simulink library "MinSegLibrary_MinSegMega"  (R2015b)
settings: Solver=ode45  StartTime=0.0  StopTime=10.0  RelTol=1e-3
libraries: arduinolib x2
settings Model: Creator=hurstj  LastModifiedBy=Administrator
settings DataIOCC: SaveFormat=Array
settings DebuggingCC: UnderspecifiedInitializationDetection=Classic  MergeDetectMultiDrivingBlocksExec=none  SolverPrmCheckMsg=warning  StateNameClashWarn=warning
settings HardwareCC: ProdBitPerPointer=32  ProdLargestAtomicFloat=None  ProdIntDivRoundTo=Undefined  ProdEndianess=Unspecified  ProdWordSize=32  ProdHWDeviceType=32-bit Generic
settings GRTTargetCC: GeneratePreprocessorConditionals=Disable all
settings ConfigComp: CovModelRefEnable=Off

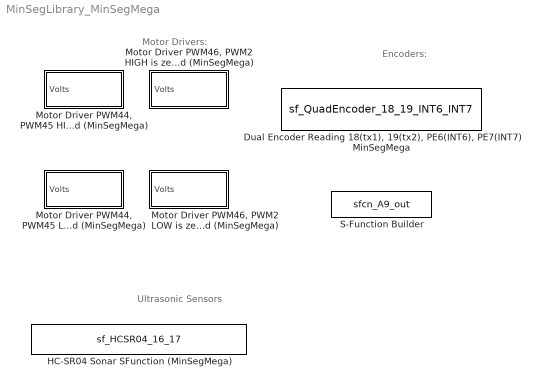
== system MinSegLibrary_MinSegMega ==
  note: Motor Drivers:
  note: Ultrasonic Sensors
  note: Encoders:
  "Dual Encoder Reading 18(tx1), 19(tx2), PE6(INT6), PE7(INT7) MinSegMega " : S-Function  InitFcn=try, set_param(gcb,'FunctionName','sf_QuadEncoder_18_19_INT6_INT7'), end  FunctionName=sf_QuadEncoder_18_19_INT6_INT7  Parameters=uint8([0 1]),uint8([18 6]),uint8([19 7])  SFunctionModules=sf_QuadEncoder_18_19_INT6_INT7_wrapper  SFunctionDeploymentMode=off  EnableBusSupport=off  mask(S-Function Builder){}
      mask init:
      | val = [[.9  0.75 0.75 1 1 .9 .9 1]',[1 1 0.75 0.75 .9 .9 1 .9]'];try , sys = get_param(gcb,'SfunBuilderFcnName');if isempty(sys), sys = get_param(gcb,'FunctionName'); end,catch, sys = get_param(gcb,'FunctionName'); end
      settings: CopyFcn=set_param(gcbh,'LinkStatus','none')  PreSaveFcn=try, set_param(gcb,'FunctionName','sf_QuadEncoder_18_19_INT6_INT7'), end  OpenFcn=sfunctionwizard(gcbh)
      mask Display: plot(val(:,1),val(:,2)),disp(sys), port_label('output',1,'pos1'), port_label('output',2,'pos2')
  HC-SR04 Sonar SFunction (MinSegMega) : S-Function  InitFcn=try, set_param(gcb,'FunctionName','sf_HCSR04_16_17'), end  FunctionName=sf_HCSR04_16_17  SFunctionModules=sf_HCSR04_16_17_wrapper  SFunctionDeploymentMode=off  EnableBusSupport=off  mask(S-Function Builder){}
      mask help: Simulink:masks:SFunctionBuilder_MD
      mask init: same as MinSegLibrary_MinSegMega/Dual Encoder Reading 18(tx1), 19(tx2), PE6(INT6), PE7(INT7) MinSegMega 
      settings: CopyFcn=set_param(gcbh,'LinkStatus','none')  PreSaveFcn=try, set_param(gcb,'FunctionName','sf_HCSR04_16_17'), end  OpenFcn=sfunctionwizard(gcbh)
      mask Display: plot(val(:,1),val(:,2)),disp(sys), port_label('output',1,'distance_cm')
  "Motor Driver PWM44, PWM45 HIGH is zero speed (MinSegMega)" : Subsystem
  "Motor Driver PWM44, PWM45 LOW is zero speed (MinSegMega)" : Subsystem
  "Motor Driver PWM46, PWM2 HIGH is zero speed (MinSegMega)" : Subsystem
  "Motor Driver PWM46, PWM2 LOW is zero speed (MinSegMega)" : Subsystem
  S-Function Builder : S-Function  InitFcn=try, set_param(gcb,'FunctionName','sfcn_A9_out'), end  FunctionName=sfcn_A9_out  Parameters=uint8(9)  SFunctionModules=sfcn_A9_out_wrapper  SFunctionDeploymentMode=off  EnableBusSupport=off  mask(S-Function Builder){}
      mask init: same as MinSegLibrary_MinSegMega/Dual Encoder Reading 18(tx1), 19(tx2), PE6(INT6), PE7(INT7) MinSegMega 
      settings: CopyFcn=set_param(gcbh,'LinkStatus','none')  PreSaveFcn=try, set_param(gcb,'FunctionName','sfcn_A9_out'), end  OpenFcn=sfunctionwizard(gcbh)
      mask Display: plot(val(:,1),val(:,2)),disp(sys), port_label('input',1,'in')

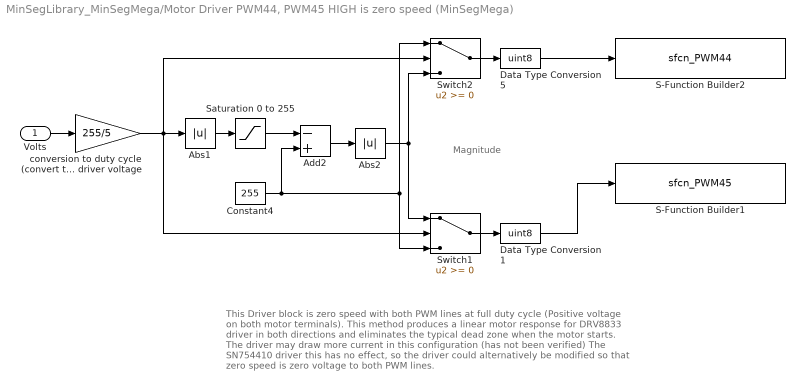
== system MinSegLibrary_MinSegMega/Motor Driver PWM44, PWM45 HIGH is zero speed (MinSegMega) ==
  note: Magnitude
  note: This Driver block is zero speed with both PWM lines at full duty cycle
      |  (Positive voltage on both motor terminals).
      | This method produces a linear motor response for DRV8833 driver
      |  in both directions and eliminates
      | the typical dead zone when the motor starts.
      | The driver may draw more current in this configuration (has not been verified)
      |
      | The SN754410 driver this has no effect, so the driver could alternatively
      | be modified so that zero speed is zero voltage to both PWM lines.
  Volts : Inport
  Abs1 : Abs
  Abs2 : Abs
  Add2 : Sum  Inputs=-+
  Constant4 : Constant  Value=255
  Data Type Conversion1 : DataTypeConversion  OutDataTypeStr=uint8
  Data Type Conversion5 : DataTypeConversion  OutDataTypeStr=uint8
  S-Function Builder1 : S-Function  InitFcn=try, set_param(gcb,'FunctionName','sfcn_PWM45'), end  FunctionName=sfcn_PWM45  Parameters=uint8(45)  SFunctionModules=sfcn_PWM45_wrapper  SFunctionDeploymentMode=off  EnableBusSupport=off  mask(S-Function Builder){}
      mask init: same as MinSegLibrary_MinSegMega/Dual Encoder Reading 18(tx1), 19(tx2), PE6(INT6), PE7(INT7) MinSegMega 
      settings: CopyFcn=set_param(gcbh,'LinkStatus','none')  PreSaveFcn=try, set_param(gcb,'FunctionName','sfcn_PWM45'), end  OpenFcn=sfunctionwizard(gcbh)
      mask Display: plot(val(:,1),val(:,2)),disp(sys), port_label('input',1,'in')
  S-Function Builder2 : S-Function  InitFcn=try, set_param(gcb,'FunctionName','sfcn_PWM44'), end  FunctionName=sfcn_PWM44  Parameters=uint8(44)  SFunctionModules=sfcn_PWM44_wrapper  SFunctionDeploymentMode=off  EnableBusSupport=off  mask(S-Function Builder){}
      mask init: same as MinSegLibrary_MinSegMega/Dual Encoder Reading 18(tx1), 19(tx2), PE6(INT6), PE7(INT7) MinSegMega 
      settings: CopyFcn=set_param(gcbh,'LinkStatus','none')  PreSaveFcn=try, set_param(gcb,'FunctionName','sfcn_PWM44'), end  OpenFcn=sfunctionwizard(gcbh)
      mask Display: plot(val(:,1),val(:,2)),disp(sys), port_label('input',1,'in')
  Saturation 0 to 255 : Saturate  UpperLimit=255  LowerLimit=0
  Switch1 : Switch
  Switch2 : Switch
  conversion to duty cycle (convert to int) denominator is motor driver voltage : Gain  Gain=255/5  OutDataTypeStr=int16
  wires:
  Data Type Conversion1/1 -> S-Function Builder1/1
  Data Type Conversion5/1 -> S-Function Builder2/1
  Switch1/1 -> Data Type Conversion1/1
  Switch2/1 -> Data Type Conversion5/1
  Abs2/1 -> Switch1/1, Switch2/3
  Add2/1 -> Abs2/1
  Constant4/1 -> Add2/2, Switch2/1, Switch1/3
  Abs1/1 -> Saturation 0 to 255/1
  Saturation 0 to 255/1 -> Add2/1
  conversion to duty cycle (convert to int) denominator is motor driver voltage/1 -> Switch1/2, Switch2/2, Abs1/1
  Volts/1 -> conversion to duty cycle (convert to int) denominator is motor driver voltage/1

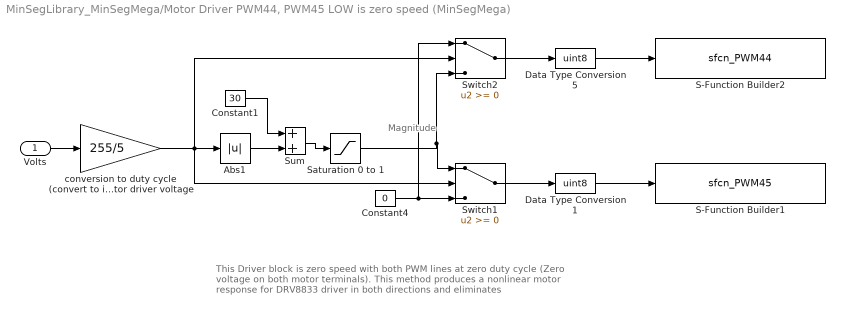
== system MinSegLibrary_MinSegMega/Motor Driver PWM44, PWM45 LOW is zero speed (MinSegMega) ==
  note: This Driver block is zero speed with both PWM lines at zero duty cycle
      |  (Zero voltage on both motor terminals).
      | This method produces a nonlinear motor response for DRV8833 driver
      |  in both directions and eliminates
  note: Magnitude
  Volts : Inport
  Abs1 : Abs
  Constant1 : Constant  Value=30
  Constant4 : Constant  Value=0
  Data Type Conversion1 : DataTypeConversion  OutDataTypeStr=uint8
  Data Type Conversion5 : DataTypeConversion  OutDataTypeStr=uint8
  S-Function Builder1 : S-Function  InitFcn=try, set_param(gcb,'FunctionName','sfcn_PWM45'), end  FunctionName=sfcn_PWM45  Parameters=uint8(45)  SFunctionModules=sfcn_PWM45_wrapper  SFunctionDeploymentMode=off  EnableBusSupport=off  mask(S-Function Builder){}
      mask init: same as MinSegLibrary_MinSegMega/Dual Encoder Reading 18(tx1), 19(tx2), PE6(INT6), PE7(INT7) MinSegMega 
      settings: CopyFcn=set_param(gcbh,'LinkStatus','none')  PreSaveFcn=try, set_param(gcb,'FunctionName','sfcn_PWM45'), end  OpenFcn=sfunctionwizard(gcbh)
      mask Display: plot(val(:,1),val(:,2)),disp(sys), port_label('input',1,'in')
  S-Function Builder2 : S-Function  InitFcn=try, set_param(gcb,'FunctionName','sfcn_PWM44'), end  FunctionName=sfcn_PWM44  Parameters=uint8(44)  SFunctionModules=sfcn_PWM44_wrapper  SFunctionDeploymentMode=off  EnableBusSupport=off  mask(S-Function Builder){}
      mask init: same as MinSegLibrary_MinSegMega/Dual Encoder Reading 18(tx1), 19(tx2), PE6(INT6), PE7(INT7) MinSegMega 
      settings: CopyFcn=set_param(gcbh,'LinkStatus','none')  PreSaveFcn=try, set_param(gcb,'FunctionName','sfcn_PWM44'), end  OpenFcn=sfunctionwizard(gcbh)
      mask Display: plot(val(:,1),val(:,2)),disp(sys), port_label('input',1,'in')
  Saturation 0 to 1 : Saturate  UpperLimit=255  LowerLimit=0
  Sum : Sum
  Switch1 : Switch
  Switch2 : Switch
  conversion to duty cycle (convert to int) denominator is motor driver voltage : Gain  Gain=255/5  OutDataTypeStr=int16
  wires:
  Volts/1 -> conversion to duty cycle (convert to int) denominator is motor driver voltage/1
  conversion to duty cycle (convert to int) denominator is motor driver voltage/1 -> Switch1/2, Abs1/1, Switch2/2
  Constant4/1 -> Switch2/1, Switch1/3
  Saturation 0 to 1/1 -> Switch2/3, Switch1/1
  Switch2/1 -> Data Type Conversion5/1
  Switch1/1 -> Data Type Conversion1/1
  Data Type Conversion5/1 -> S-Function Builder2/1
  Data Type Conversion1/1 -> S-Function Builder1/1
  Abs1/1 -> Sum/2
  Sum/1 -> Saturation 0 to 1/1
  Constant1/1 -> Sum/1

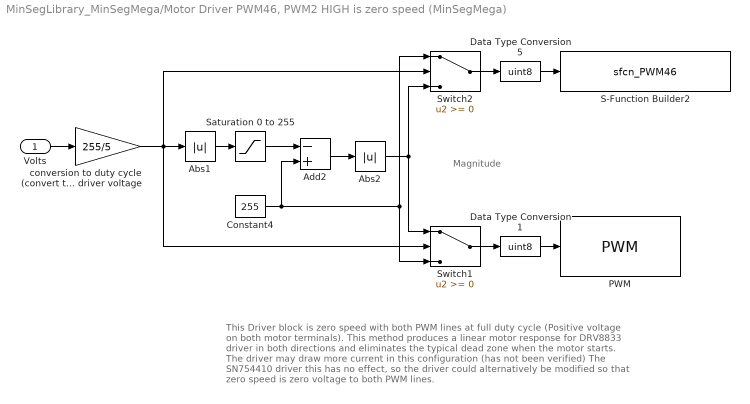
== system MinSegLibrary_MinSegMega/Motor Driver PWM46, PWM2 HIGH is zero speed (MinSegMega) ==
  note: Magnitude
  note: This Driver block is zero speed with both PWM lines at full duty cycle
      |  (Positive voltage on both motor terminals).
      | This method produces a linear motor response for DRV8833 driver
      |  in both directions and eliminates
      | the typical dead zone when the motor starts.
      | The driver may draw more current in this configuration (has not been verified)
      |
      | The SN754410 driver this has no effect, so the driver could alternatively
      | be modified so that zero speed is zero voltage to both PWM lines.
  Volts : Inport
  Abs1 : Abs
  Abs2 : Abs
  Add2 : Sum  Inputs=-+
  Constant4 : Constant  Value=255
  Data Type Conversion1 : DataTypeConversion  OutDataTypeStr=uint8
  Data Type Conversion5 : DataTypeConversion  OutDataTypeStr=uint8
  PWM : arduinolib/PWM  pinNumber=2
  S-Function Builder2 : S-Function  InitFcn=try, set_param(gcb,'FunctionName','sfcn_PWM46'), end  FunctionName=sfcn_PWM46  Parameters=uint8(46)  SFunctionModules=sfcn_PWM46_wrapper  SFunctionDeploymentMode=off  EnableBusSupport=off  mask(S-Function Builder){}
      mask init: same as MinSegLibrary_MinSegMega/Dual Encoder Reading 18(tx1), 19(tx2), PE6(INT6), PE7(INT7) MinSegMega 
      settings: CopyFcn=set_param(gcbh,'LinkStatus','none')  PreSaveFcn=try, set_param(gcb,'FunctionName','sfcn_PWM46'), end  OpenFcn=sfunctionwizard(gcbh)
      mask Display: plot(val(:,1),val(:,2)),disp(sys), port_label('input',1,'in')
  Saturation 0 to 255 : Saturate  UpperLimit=255  LowerLimit=0
  Switch1 : Switch
  Switch2 : Switch
  conversion to duty cycle (convert to int) denominator is motor driver voltage : Gain  Gain=255/5  OutDataTypeStr=int16
  wires:
  Data Type Conversion1/1 -> PWM/1
  Data Type Conversion5/1 -> S-Function Builder2/1
  Switch1/1 -> Data Type Conversion1/1
  Switch2/1 -> Data Type Conversion5/1
  Abs2/1 -> Switch1/1, Switch2/3
  Add2/1 -> Abs2/1
  Constant4/1 -> Add2/2, Switch2/1, Switch1/3
  Abs1/1 -> Saturation 0 to 255/1
  Saturation 0 to 255/1 -> Add2/1
  conversion to duty cycle (convert to int) denominator is motor driver voltage/1 -> Switch1/2, Switch2/2, Abs1/1
  Volts/1 -> conversion to duty cycle (convert to int) denominator is motor driver voltage/1

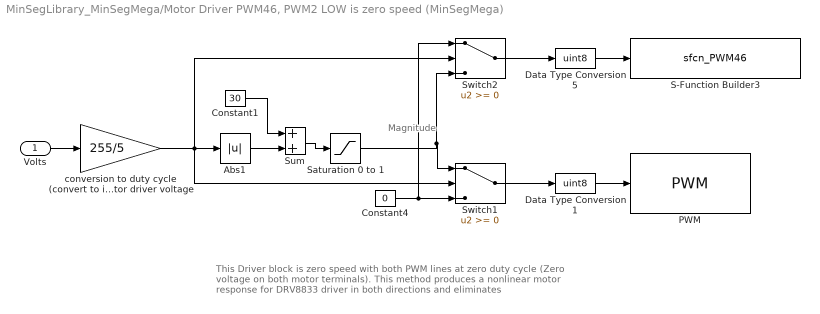
== system MinSegLibrary_MinSegMega/Motor Driver PWM46, PWM2 LOW is zero speed (MinSegMega) ==
  note: This Driver block is zero speed with both PWM lines at zero duty cycle
      |  (Zero voltage on both motor terminals).
      | This method produces a nonlinear motor response for DRV8833 driver
      |  in both directions and eliminates
  note: Magnitude
  Volts : Inport
  Abs1 : Abs
  Constant1 : Constant  Value=30
  Constant4 : Constant  Value=0
  Data Type Conversion1 : DataTypeConversion  OutDataTypeStr=uint8
  Data Type Conversion5 : DataTypeConversion  OutDataTypeStr=uint8
  PWM : arduinolib/PWM  pinNumber=2
  S-Function Builder3 : S-Function  InitFcn=try, set_param(gcb,'FunctionName','sfcn_PWM46'), end  FunctionName=sfcn_PWM46  Parameters=uint8(46)  SFunctionModules=sfcn_PWM46_wrapper  SFunctionDeploymentMode=off  EnableBusSupport=off  mask(S-Function Builder){}
      mask init: same as MinSegLibrary_MinSegMega/Dual Encoder Reading 18(tx1), 19(tx2), PE6(INT6), PE7(INT7) MinSegMega 
      settings: CopyFcn=set_param(gcbh,'LinkStatus','none')  PreSaveFcn=try, set_param(gcb,'FunctionName','sfcn_PWM46'), end  OpenFcn=sfunctionwizard(gcbh)
      mask Display: plot(val(:,1),val(:,2)),disp(sys), port_label('input',1,'in')
  Saturation 0 to 1 : Saturate  UpperLimit=255  LowerLimit=0
  Sum : Sum
  Switch1 : Switch
  Switch2 : Switch
  conversion to duty cycle (convert to int) denominator is motor driver voltage : Gain  Gain=255/5  OutDataTypeStr=int16
  wires:
  Volts/1 -> conversion to duty cycle (convert to int) denominator is motor driver voltage/1
  conversion to duty cycle (convert to int) denominator is motor driver voltage/1 -> Switch1/2, Abs1/1, Switch2/2
  Constant4/1 -> Switch2/1, Switch1/3
  Saturation 0 to 1/1 -> Switch2/3, Switch1/1
  Switch2/1 -> Data Type Conversion5/1
  Switch1/1 -> Data Type Conversion1/1
  Data Type Conversion5/1 -> S-Function Builder3/1
  Data Type Conversion1/1 -> PWM/1
  Abs1/1 -> Sum/2
  Sum/1 -> Saturation 0 to 1/1
  Constant1/1 -> Sum/1
